simulink model "compensador_en_bluepill"  (R2021a)
settings: Solver=VariableStepAuto  StartTime=0.0  StopTime=1  RelTol=1e-3
libraries: instrumentseriallib x3
settings Model: Creator=Nancy  LastModifiedBy=Nano

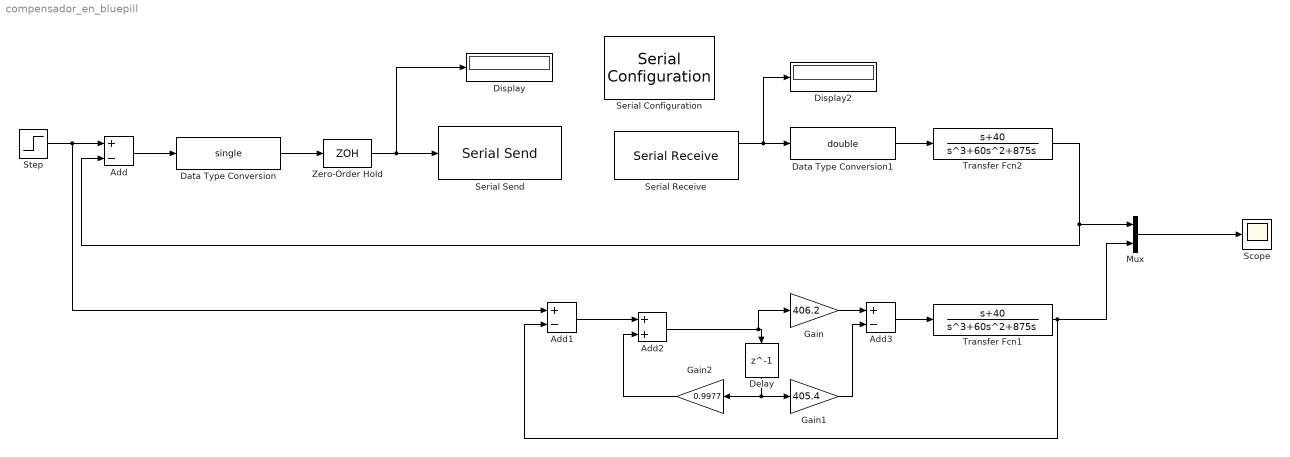
== system compensador_en_bluepill ==
  Add : Sum  Inputs=+-  AccumDataTypeStr=single  OutDataTypeStr=single
  Add1 : Sum  Inputs=+-  AccumDataTypeStr=double  OutDataTypeStr=double
  Add2 : Sum  AccumDataTypeStr=double  OutDataTypeStr=double
  Add3 : Sum  Inputs=+-  AccumDataTypeStr=double  OutDataTypeStr=double
  Data Type Conversion : DataTypeConversion  OutDataTypeStr=single
  Data Type Conversion1 : DataTypeConversion  OutDataTypeStr=double  LockScale=on
  Delay : Delay  DelayLength=1  InitialCondition=0
  Display : Display
      settings: Format=hex (Stored Integer)
  Display2 : Display
      settings: Format=hex (Stored Integer)
  Gain : Gain  Gain=406.2  OutDataTypeStr=double
  Gain1 : Gain  Gain=405.4  OutDataTypeStr=double
  Gain2 : Gain  Gain=0.9977  OutDataTypeStr=double
  Mux : Mux  Inputs=2
  Scope : Scope
  Serial Configuration : instrumentseriallib/Serial Configuration  Priority=-200000  Port=COM5  ComPort=COM5  BaudRate=115200  DataBits=8  Parity=none  StopBits=1  ByteOrder=little-endian  FlowControl=none  Timeout=100  SimulateUsing=Interpreted execution  BlockInModel=on
  Serial Receive : instrumentseriallib/Serial Receive  Priority=1  Port=COM5  ComPort=COM5  DataType=single  SaveDataType=uint8  ToggleHeader=off  Header=[]  ToggleTerminator=off  Terminator=<none>  CustomTerminator=[]  ToggleDataSize=on  DataSize=[1 1]  EnableBlockingMode=off  ActionDataUnavailable=Output last received value  ActionWhenDataUnavailable=Output last received value  CustomValue=0  SampleTime=0.0001  SimulateUsing=Interpreted execution  BlockInModel=on
  Serial Send : instrumentseriallib/Serial Send  Priority=1  Port=COM5  ComPort=COM5  Header=[]  Terminator=<none>  CustomTerminator=[]  EnableBlockingMode=off  SimulateUsing=Interpreted execution  BlockInModel=on
  Step : Step  Time=0  OutDataTypeStr=single  SampleTime=0
  Transfer Fcn1 : TransferFcn  Numerator=[1 40]  Denominator=[1 60 875 0]
  Transfer Fcn2 : TransferFcn  Numerator=[1 40]  Denominator=[1 60 875 0]
  Zero-Order Hold : ZeroOrderHold  SampleTime=0.0001
  wires:
  Serial Receive/1 -> Data Type Conversion1/1, Display2/1
  Data Type Conversion1/1 -> Transfer Fcn2/1
  Add/1 -> Data Type Conversion/1
  Transfer Fcn2/1 -> Mux/1, Add/2
  Step/1 -> Add1/1, Add/1
  Data Type Conversion/1 -> Zero-Order Hold/1
  Zero-Order Hold/1 -> Display/1, Serial Send/1
  Transfer Fcn1/1 -> Add1/2, Mux/2
  Mux/1 -> Scope/1
  Add2/1 -> Gain/1, Delay/1
  Gain/1 -> Add3/1
  Delay/1 -> Gain2/1, Gain1/1
  Gain1/1 -> Add3/2
  Gain2/1 -> Add2/2
  Add1/1 -> Add2/1
  Add3/1 -> Transfer Fcn1/1
